simulink model "periodSensor"  (R2018b)
settings: Solver=FixedStepAuto  StartTime=0.0  StopTime=500.0  FixedStep=0.01  RelTol=1e-3
values from neighbouring files (symbols this model uses):
  waveAmpTime = [t' yfin']    [makeWaveAmpTime.m]
undefined symbols (not defined in the file or in its folder): simu, waves
settings Model: Creator=glennond  LastModifiedBy=dng26

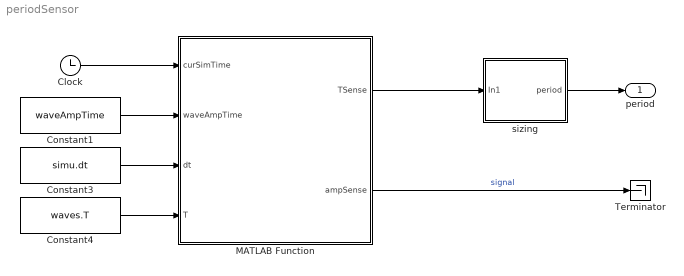
== system periodSensor ==
  Clock : Clock
  Constant1 : Constant  Value=waveAmpTime
  Constant3 : Constant  Value=simu.dt
  Constant4 : Constant  Value=waves.T
  MATLAB Function : MATLAB Function  TreatAsAtomicUnit=on  SystemSampleTime=0.1
  Terminator : Terminator
  sizing : Subsystem
  period : Outport
  wires:
  Clock/1 -> MATLAB Function/1(curSimTime)
  Constant1/1 -> MATLAB Function/2(waveAmpTime)
  Constant3/1 -> MATLAB Function/3(dt)
  MATLAB Function/2(ampSense) -> Terminator/1  "signal"
  Constant4/1 -> MATLAB Function/4(T)
  MATLAB Function/1(TSense) -> sizing/1(In1)
  sizing/1(period) -> period/1

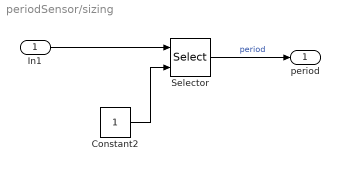
== system periodSensor/sizing ==
  In1 : Inport
  Constant2 : Constant
  Selector : Selector  InputPortWidth=2  IndexOptions=Index vector (port)  Indices=1  OutputSizes=1
  period : Outport
  wires:
  Constant2/1 -> Selector/2
  In1/1 -> Selector/1
  Selector/1 -> period/1  "period"

== matlab function periodSensor/MATLAB Function ==
  data: curSimTime input; TSense output size=[1 2]; waveAmpTime input; dt input; ampSense output; T input
function [TSense,ampSense] = getPeriod(curSimTime, waveAmpTime, dt, T)

% This function sort of pretends we don't know the full time series for
% wave amplitude since for control purposes, we won't. Use a rolling sample
% window of the wave height and DFT to get an approximate period for
% input into the controller. This way the control can respond to a more
% "instantaneous" value for period. In some instances we may need to
% "cheat" and access Waves.T, or the entire series, in order to pick a
% default value. A more realistic suitable default value might be
% a known average period for a given location / season / time of day.

% REQUIREMENTS: - a fixed step simulation (simu.solver = 'ode4'; simu.dt = defined)
% does not support etaImport waveclass (need a default Waves.T, could be
% made to support this)

% Inputs: 
% curSimTime: the current simulation time
% waveAmpTime: the wave aplitude timeseries
% dt: simulation step
% T: default wave period

% Outputs
% Tsense: approximate period
% sig: current amp value


if curSimTime == 0 % pre-historic...
    TSense = T;
    ampSense = 0;
else
    
    t = waveAmpTime(:,1);
    amp = waveAmpTime(:,2);

    % Time series of amplitudes from simulation start to current time step
    allPastt = t(t <= curSimTime);
    allPastSamples = numel(allPastt);
    allPastAmp = amp(1:allPastSamples);
    
    % Current Amplitude
    ampSense = allPastAmp(end);

    % Create a 5-ish cycle sample window
    samplesPerCycle = T/dt;
    if curSimTime < 5*T
        windowSamples = allPastSamples; % use what we got
    else
        windowSamples = 5*samplesPerCycle;
    end

    windowPastt = allPastt(end-windowSamples+1:end);
    windowPastAmp = allPastAmp(end-windowSamples+1:end);

    % Sampling frequency
    fs = 1/dt;

    %Signal Length
    L = windowSamples;

    % Calculate fft
    ampDftMags = abs(fft(windowPastAmp));

    %%Single-sided magnitude spectrum with frequency axis in Hertz
    % Each bin frequency is separated by fs/L Hertz.
    binVals = [0 : L-1];
    fHz = binVals*fs/L;
    L_2 = ceil(L/2);

    freqs = fHz(1:L_2);
    mags = ampDftMags(1:L_2);

    [~, dPd] = max(mags);
    TSense = 1/freqs(dPd);


    if TSense == Inf
       TSense = T;
    end
end
end
